simulink model "MultipleModule_SpeedTorqueConfiguration"  (R2016a)
settings: Solver=VariableStepAuto  StartTime=0.0  StopTime=0.5  RelTol=1e-3
undefined symbols (not defined in the file or in its folder): DCVolt, freq
libraries: powerlib x11, powerlib_meascontrol x11, dspstat3 x1
settings Model: Creator=kkfrk  LastModifiedBy=ugurm

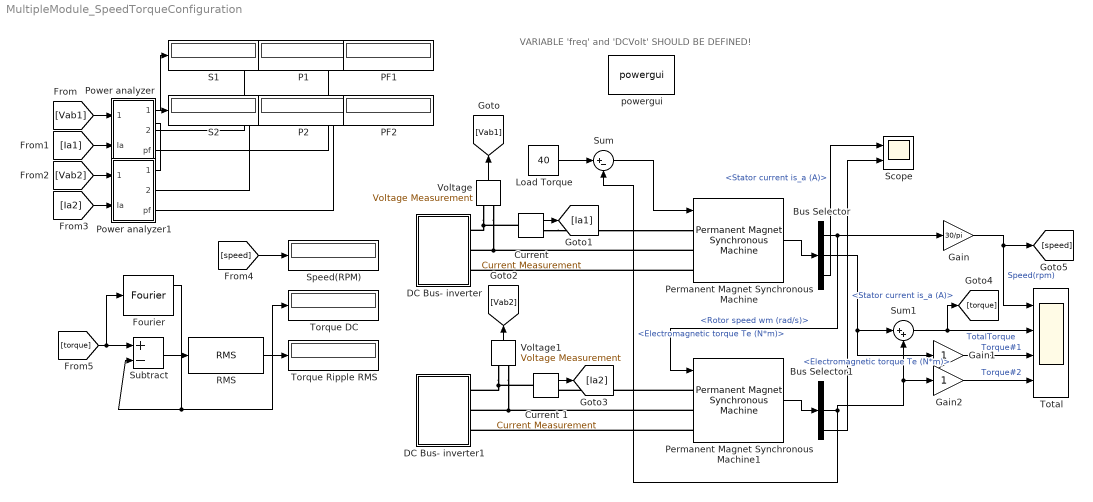
== system MultipleModule_SpeedTorqueConfiguration ==
  note: VARIABLE 'freq' and 'DCVolt' SHOULD BE DEFINED!
  Bus Selector : BusSelector  OutputSignals=Rotor speed wm (rad/s),Electromagnetic torque Te (N*m),Stator current is_a (A)
  Bus Selector1 : BusSelector  OutputSignals=Rotor speed wm (rad/s),Electromagnetic torque Te (N*m),Stator current is_a (A)
  Current : powerlib/Measurements/Current Measurement  PhasorSimulation=off  OutputType=Complex  PSBequivalent=0
  Current 1 : powerlib/Measurements/Current Measurement  PhasorSimulation=off  OutputType=Complex  PSBequivalent=0
  DC Bus- inverter : Subsystem
  DC Bus- inverter1 : Subsystem
  Fourier : powerlib_meascontrol/Measurements/Fourier  Freq=freq  n=0  InInit=[0, 0]  Ts=0
  Gain : Gain  Gain=30/pi
  Gain1 : Gain
  Gain2 : Gain
  Load Torque : Constant  Value=40
  P1 : Display
  P2 : Display
  PF1 : Display
  PF2 : Display
  Permanent Magnet Synchronous Machine : powerlib/Machines/Permanent Magnet Synchronous Machine  NbPhases=3  FluxDistribution=Sinusoidal  RotorType=Round  MechanicalLoad=Torque Tm  PresetModel=No  ShowDetailedParameters=on  MeasurementBus=off  Resistance=0.10389  Inductance=8.5e-3  dqInductances=[8.5e-3,8.5e-3]  La=0.00020966  MachineConstant=Flux linkage established by magnets (V.s)  Flux=0.01204  VoltageCst=10.9191  TorqueCst=0.0903  Flat=120  Mechanical=[5.3476e-05 0.00016761 5]  PolePairs=4  InitialConditions=[0,0, 0,0]  InitialConditions5ph=[0 0 0 0 0 0]  TsPowergui=0  TsBlock=-1  RefAngle=90 degrees behind phase A axis (modified Park)
  Permanent Magnet Synchronous Machine1 : powerlib/Machines/Permanent Magnet Synchronous Machine  NbPhases=3  FluxDistribution=Sinusoidal  RotorType=Round  MechanicalLoad=Speed w  PresetModel=No  ShowDetailedParameters=on  MeasurementBus=off  Resistance=0.10389  Inductance=8.5e-3  dqInductances=[8.5e-3,8.5e-3]  La=0.00020966  MachineConstant=Flux linkage established by magnets (V.s)  Flux=0.01204  VoltageCst=10.9191  TorqueCst=0.0903  Flat=120  Mechanical=[5.3476e-05 0.00016761 5]  PolePairs=5  InitialConditions=[0,0, 0,0]  InitialConditions5ph=[0 0 0 0 0 0]  TsPowergui=0  TsBlock=-1  RefAngle=90 degrees behind phase A axis (modified Park)
  Power analyzer : Subsystem  RequirementInfo={} %GIDa_ceeed5ee_c572_4f23_9706_eea9f63106ff
  Power analyzer1 : Subsystem  RequirementInfo={} %GIDa_3bdbdf9c_be24_4f92_baa2_c843eb9c092a
  RMS : dspstat3/RMS  run=off  reset_popup=None  InputProcessing=Columns as channels (frame based)  directionMode=Each column  dimension=1
  S1 : Display
  S2 : Display
  Scope : Scope  NumInputPorts=2
  Speed(RPM) : Display
  Subtract : Sum  Inputs=+-
  Sum : Sum  Inputs=|+-
  Sum1 : Sum  Inputs=|++
  Torque DC : Display
  Torque Ripple RMS : Display
  Total : Scope  NumInputPorts=4
  Voltage : powerlib/Measurements/Voltage Measurement  PhasorSimulation=off  OutputType=Complex  PSBequivalent=0
  Voltage1 : powerlib/Measurements/Voltage Measurement  PhasorSimulation=off  OutputType=Complex  PSBequivalent=0
  powergui : powerlib/powergui  Priority=1  SimulationMode=Discrete  SolverType=Tustin/Backward Euler (TBE)  SampleTime=1e-6  frequency=60  SPID=off  DisableSnubberDevices=off  DisableRonSwitches=off  DisableVfSwitches=off  SwTol=0  DisplayEquations=off  Interpol=off  ExternalGateDelay=off  methode=off  Ts=10  FunctionMessages=off  echomessages=off  HookPort=off  EnableUseOfTLC=off  x0status=blocks  frequencyindice=0  Pbase=100e6  ErrMax=1e-4  Iterations=50  UnitsV=kV  UnitsW=MW  buscounter=0  RestoreLinks=warning  ResistiveCurrentMeasurement=off  Frange=[0:2:500]  Ylog=off  Xlog=on  ShowGrid=off  save=off  variable=ZData  structure=0  ZoomFFT=off  StartTime=0.0  cycles=1  DisplayStyle=1  fundamental=60  FreqAxis=off  MaxFrequency=1000  frequencyindicesteady=1  RmsSteady=1  display=off
  wires:
  Permanent Magnet Synchronous Machine/1 -> Bus Selector/1
  Bus Selector/1 -> Permanent Magnet Synchronous Machine1/1, Gain/1  "<Rotor speed wm (rad/s)>"
  Permanent Magnet Synchronous Machine1/1 -> Bus Selector1/1
  Bus Selector1/2 -> Sum/2, Gain2/1, Sum1/2  "<Electromagnetic torque Te (N*m)>"
  Load Torque/1 -> Sum/1
  Sum/1 -> Permanent Magnet Synchronous Machine/1
  Voltage/1 -> [Vab1]
  Current/1 -> [Ia1]
  Voltage1/1 -> [Vab2]
  Current 1/1 -> [Ia2]
  [Vab1] -> Power analyzer/1(Vab)
  [Ia1] -> Power analyzer/2(Ia)
  [Vab2] -> Power analyzer1/1(Vab)
  [Ia2] -> Power analyzer1/2(Ia)
  Power analyzer/1(Sin) -> S1/1
  Power analyzer/2(Pin) -> P1/1
  Power analyzer/3(pf) -> PF1/1
  Power analyzer1/1(Sin) -> S2/1
  Power analyzer1/2(Pin) -> P2/1
  Power analyzer1/3(pf) -> PF2/1
  Bus Selector/2 -> Gain1/1, Sum1/1  "<Electromagnetic torque Te (N*m)>"
  Sum1/1 -> [torque], Total/2  "TotalTorque"
  Gain1/1 -> Total/3  "Torque#1"
  Gain2/1 -> Total/4  "Torque#2"
  Bus Selector/3 -> Scope/1  "<Stator current is_a (A)>"
  Bus Selector1/3 -> Scope/2  "<Stator current is_a (A)>"
  Gain/1 -> [speed], Total/1  "Speed(rpm)"
  Fourier/1 -> Torque DC/1, Subtract/2
  Subtract/1 -> RMS/1
  RMS/1 -> Torque Ripple RMS/1
  [speed] -> Speed(RPM)/1
  [torque] -> Subtract/1, Fourier/1
  connections:
  Voltage/LConn1 -- Current/LConn1 -- DC Bus- inverter/RConn1
  Voltage/LConn2 -- Permanent Magnet Synchronous Machine/LConn2 -- DC Bus- inverter/RConn2
  Current/RConn1 -- Permanent Magnet Synchronous Machine/LConn1
  Permanent Magnet Synchronous Machine/LConn3 -- DC Bus- inverter/RConn3
  Voltage1/LConn1 -- Current 1/LConn1 -- DC Bus- inverter1/RConn1
  Voltage1/LConn2 -- Permanent Magnet Synchronous Machine1/LConn2 -- DC Bus- inverter1/RConn2
  Permanent Magnet Synchronous Machine1/LConn3 -- DC Bus- inverter1/RConn3
  Permanent Magnet Synchronous Machine1/LConn1 -- Current 1/RConn1

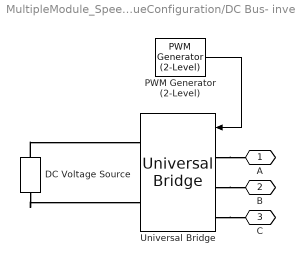
== system MultipleModule_SpeedTorqueConfiguration/DC Bus- inverter ==
  DC Voltage Source : powerlib/Electrical Sources/DC Voltage Source  Amplitude=DCVolt  Measurements=None
  PWM Generator (2-Level) : powerlib_meascontrol/Pulse & Signal Generators/PWM Generator (2-Level)  ModulatorType=Three-phase bridge (6 pulses)  ModulatorMode=Unsynchronized  Fc=27*freq  Pc=90  nF=27  MinMax="[ -1  1 ]"  SamplingTechnique=Natural  ModulatingSignals=on  m=0.8  Freq=freq  Phase=0  Ts=0  ShowCarrierOutport=off
  Universal Bridge : powerlib/Power Electronics/Universal Bridge  Arms=3  SnubberResistance=1e5  SnubberCapacitance=inf  Device=IGBT / Diodes  Ron=1e-3  Lon=0  ForwardVoltages="[  0  0  ]"  ForwardVoltage=0  GTOparameters=[ 10e-6 , 20e-6 ]  IGBTparameters=[ 1e-6 , 2e-6 ]  Measurements=None  Measurements_2=None  converterType=Rectifier
  A : PMIOPort  Port=1  Side=Right
  B : PMIOPort  Port=2  Side=Right
  C : PMIOPort  Port=3  Side=Right
  wires:
  PWM Generator (2-Level)/1 -> Universal Bridge/1
  connections:
  Universal Bridge/LConn2 -- B/RConn1
  Universal Bridge/LConn3 -- C/RConn1
  Universal Bridge/LConn1 -- A/RConn1
  DC Voltage Source/LConn1 -- Universal Bridge/RConn2
  DC Voltage Source/RConn1 -- Universal Bridge/RConn1

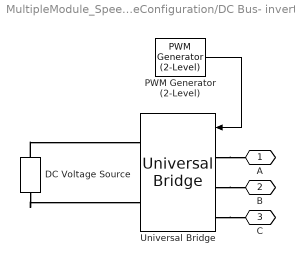
== system MultipleModule_SpeedTorqueConfiguration/DC Bus- inverter1 ==
  DC Voltage Source : powerlib/Electrical Sources/DC Voltage Source  Amplitude=DCVolt  Measurements=None
  PWM Generator (2-Level) : powerlib_meascontrol/Pulse & Signal Generators/PWM Generator (2-Level)  ModulatorType=Three-phase bridge (6 pulses)  ModulatorMode=Unsynchronized  Fc=27*freq  Pc=90  nF=27  MinMax="[ -1  1 ]"  SamplingTechnique=Natural  ModulatingSignals=on  m=0.8  Freq=freq  Phase=0  Ts=0  ShowCarrierOutport=off
  Universal Bridge : powerlib/Power Electronics/Universal Bridge  Arms=3  SnubberResistance=1e5  SnubberCapacitance=inf  Device=IGBT / Diodes  Ron=1e-3  Lon=0  ForwardVoltages="[  0  0  ]"  ForwardVoltage=0  GTOparameters=[ 10e-6 , 20e-6 ]  IGBTparameters=[ 1e-6 , 2e-6 ]  Measurements=None  Measurements_2=None  converterType=Rectifier
  A : PMIOPort  Port=1  Side=Right
  B : PMIOPort  Port=2  Side=Right
  C : PMIOPort  Port=3  Side=Right
  wires:
  PWM Generator (2-Level)/1 -> Universal Bridge/1
  connections:
  Universal Bridge/LConn2 -- B/RConn1
  Universal Bridge/LConn3 -- C/RConn1
  Universal Bridge/LConn1 -- A/RConn1
  DC Voltage Source/LConn1 -- Universal Bridge/RConn2
  DC Voltage Source/RConn1 -- Universal Bridge/RConn1

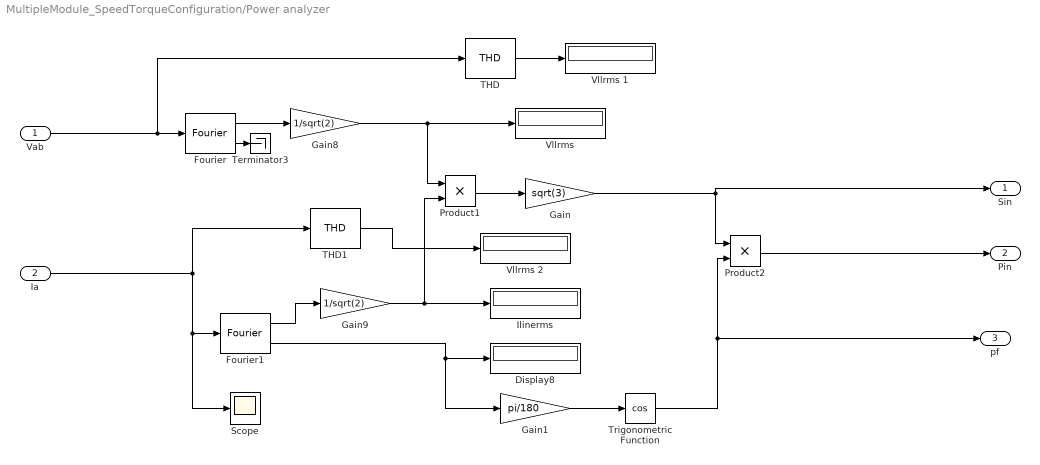
== system MultipleModule_SpeedTorqueConfiguration/Power analyzer ==
  Vab : Inport
  Ia : Inport  Port=2
  Display8 : Display
  Fourier : powerlib_meascontrol/Measurements/Fourier  Freq=freq  n=1  InInit=[0, 0]  Ts=0
  Fourier1 : powerlib_meascontrol/Measurements/Fourier  Freq=freq  n=1  InInit=[0, 0]  Ts=0
  Gain : Gain  Gain=sqrt(3)
  Gain1 : Gain  Gain=pi/180
  Gain8 : Gain  Gain=1/sqrt(2)
  Gain9 : Gain  Gain=1/sqrt(2)
  "Ilinerms " : Display
  Product1 : Product
  Product2 : Product
  Scope : Scope
  THD : powerlib_meascontrol/Measurements/THD  Freq=freq  Ts=0
  THD1 : powerlib_meascontrol/Measurements/THD  Freq=freq  Ts=0
  Terminator3 : Terminator
  Trigonometric Function : Trigonometry  Operator=cos
  "Vllrms " : Display
  Vllrms 1 : Display
  Vllrms 2 : Display
  Sin : Outport
  Pin : Outport  Port=2
  pf : Outport  Port=3
  wires:
  Gain8/1 -> Product1/1, "Vllrms "/1
  Gain9/1 -> "Ilinerms "/1, Product1/2
  Ia/1 -> Scope/1, Fourier1/1, THD1/1
  Fourier1/1 -> Gain9/1
  Vab/1 -> THD/1, Fourier/1
  Fourier/1 -> Gain8/1
  Product1/1 -> Gain/1
  Gain/1 -> Sin/1, Product2/1
  Fourier1/2 -> Gain1/1, Display8/1
  Trigonometric Function/1 -> pf/1, Product2/2
  Gain1/1 -> Trigonometric Function/1
  Product2/1 -> Pin/1
  Fourier/2 -> Terminator3/1
  THD/1 -> Vllrms 1/1
  THD1/1 -> Vllrms 2/1

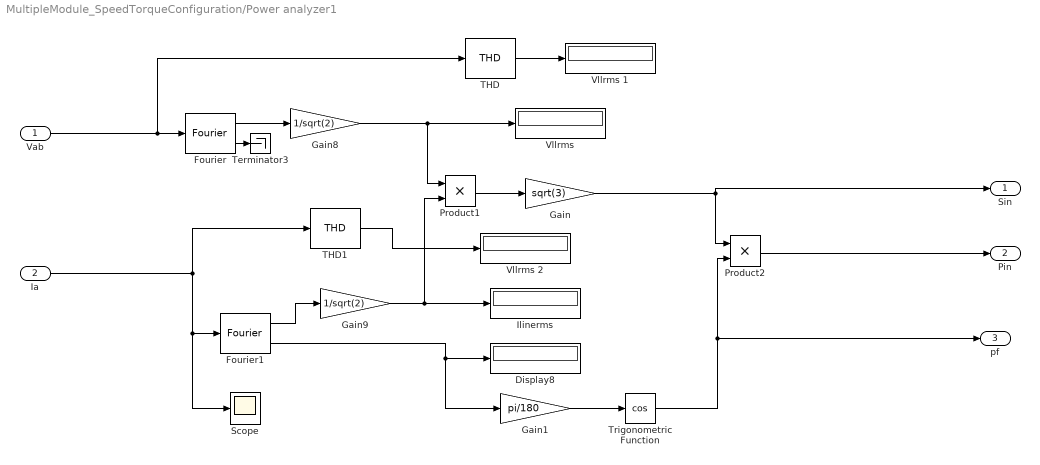
== system MultipleModule_SpeedTorqueConfiguration/Power analyzer1 ==
  Vab : Inport
  Ia : Inport  Port=2
  Display8 : Display
  Fourier : powerlib_meascontrol/Measurements/Fourier  Freq=freq  n=1  InInit=[0, 0]  Ts=0
  Fourier1 : powerlib_meascontrol/Measurements/Fourier  Freq=freq  n=1  InInit=[0, 0]  Ts=0
  Gain : Gain  Gain=sqrt(3)
  Gain1 : Gain  Gain=pi/180
  Gain8 : Gain  Gain=1/sqrt(2)
  Gain9 : Gain  Gain=1/sqrt(2)
  "Ilinerms " : Display
  Product1 : Product
  Product2 : Product
  Scope : Scope
  THD : powerlib_meascontrol/Measurements/THD  Freq=freq  Ts=0
  THD1 : powerlib_meascontrol/Measurements/THD  Freq=freq  Ts=0
  Terminator3 : Terminator
  Trigonometric Function : Trigonometry  Operator=cos
  "Vllrms " : Display
  Vllrms 1 : Display
  Vllrms 2 : Display
  Sin : Outport
  Pin : Outport  Port=2
  pf : Outport  Port=3
  wires:
  THD1/1 -> Vllrms 2/1
  THD/1 -> Vllrms 1/1
  Fourier/2 -> Terminator3/1
  Product2/1 -> Pin/1
  Gain1/1 -> Trigonometric Function/1
  Trigonometric Function/1 -> Product2/2, pf/1
  Fourier1/2 -> Display8/1, Gain1/1
  Gain/1 -> Product2/1, Sin/1
  Product1/1 -> Gain/1
  Fourier/1 -> Gain8/1
  Vab/1 -> Fourier/1, THD/1
  Fourier1/1 -> Gain9/1
  Ia/1 -> THD1/1, Fourier1/1, Scope/1
  Gain9/1 -> Product1/2, "Ilinerms "/1
  Gain8/1 -> "Vllrms "/1, Product1/1
